simulink model "Glide_slope_controller3"  (R2019b)
settings: Solver=VariableStepAuto  StartTime=0.0  StopTime=400  RelTol=1e-3
values from neighbouring files (symbols this model uses):
  A_gs = A_longitude_lo([1 3 4 2 5], [1 3 4 2 5])    [FindF16Dynamics.m]    (also in FindF16Dynamics_Chapter8.m)
  alpha = 8.49    [FindF16Dynamics.m]    (also in FindF16Dynamics_Chapter8.m = 10.4511; FindF16Dynamics_KIllian.m; trim_F16.m = alpha*pi/180)
  B_gs = A_longitude_lo([1 3 4 2 5], [6, 7])    [FindF16Dynamics.m]    (also in FindF16Dynamics_Chapter8.m)
  C_gs = C_longitude_lo([1 3 4 2 5], [1 3 4 2 5])    [FindF16Dynamics.m]    (also in FindF16Dynamics_Chapter8.m)
  D_gs = D_longitude_lo([1 3 4 2 5], [1])    [FindF16Dynamics.m]    (also in FindF16Dynamics_Chapter8.m = D_longitude_lo([1 3 4 2 5], [1, 2]))
  thrust = 5000    [FindF16Dynamics.m]    (also in FindF16Dynamics_Chapter8.m = 2826.8165; FindF16Dynamics_KIllian.m)
  velocity = 300    [FindF16Dynamics.m]    (also in FindF16Dynamics_Chapter8.m; FindF16Dynamics_KIllian.m = input('Enter the velocity for the simulation (ft/s):  '); FindF16Dynamics_Q6,7.m = 900; FindF16Dynamics_Q6-7.m = 900)
undefined symbols (not defined in the file or in its folder): d_0, Gamma_0, R_0, Slope_Ramp_Gamma, t_flare, tau
libraries: simulink x9
settings Model: Creator=tomas  LastModifiedBy=tomas
settings DebuggingCC: ArithmeticOperatorsInVariantConditions=warning
settings SFSimCC: CustomCodeUndefinedFunction=UseInterfaceOnly

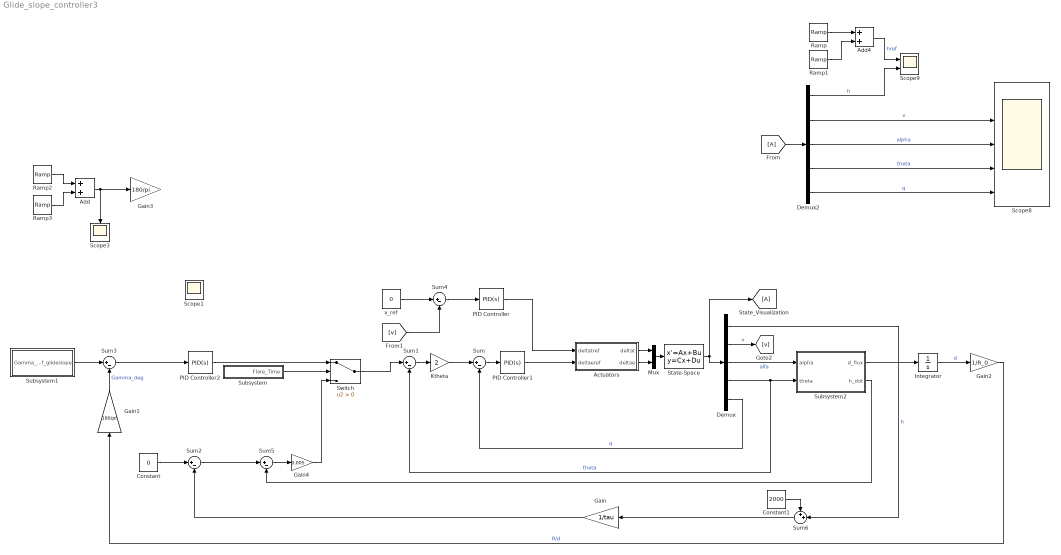
== system Glide_slope_controller3 ==
  Actuators : Subsystem
  Add : Sum
  Add4 : Sum
  Constant : Constant  Value=0
  Constant1 : Constant  Value=2000
  Demux : Demux  Outputs=5
  Demux2 : Demux  Outputs=5
  Gain : Gain  Gain=1/tau
  Gain1 : Gain  Gain=180/pi
  Gain2 : Gain  Gain=1/R_0
  Gain3 : Gain  Gain=180/pi
  Gain4 : Gain  Gain=0.005
  Integrator : Integrator  InitialCondition=d_0
  Ktheta : Gain  Gain=2
  Mux : Mux  Inputs=2
  PID Controller : simulink/Continuous/PID Controller  Controller=PID  Form=Parallel  TimeDomain=Continuous-time  SampleTime=-1  IntegratorMethod=Forward Euler  FilterMethod=Forward Euler  ControllerParametersSource=internal  P=220.313659448083  I=13.48667015583  D=-5.78338115797217  UseFilter=on  N=38.0942658680534  TunerSelectOption=Transfer Function Based (PID Tuner App)  InitialConditionSource=internal  InitialConditionForIntegrator=0  InitialConditionForFilter=0  DifferentiatorICPrevScaledInput=0  ExternalReset=none  TrackingMode=off  Kt=1  LimitOutput=off  UpperSaturationLimit=inf  LowerSaturationLimit=-inf  LinearizeAsGain=on  AntiWindupMode=none  Kb=1  POutMin=[]  POutMax=[]  IOutMin=[]  IOutMax=[]  DOutMin=[]  DOutMax=[]  NOutMin=[]  NOutMax=[]  SumOutMin=[]  SumOutMax=[]  SaturationOutMin=[]  SaturationOutMax=[]  PParamMin=[]  PParamMax=[]  IParamMin=[]  IParamMax=[]  DParamMin=[]  DParamMax=[]  NParamMin=[]  NParamMax=[]  KbParamMin=[]  KbParamMax=[]  KtParamMin=[]  KtParamMax=[]  KbOutMin=[]  KbOutMax=[]  KtOutMin=[]  KtOutMax=[]  IntegratorOutMin=[]  IntegratorOutMax=[]  FilterOutMin=[]  FilterOutMax=[]  SumI1OutMin=[]  SumI1OutMax=[]  SumI2OutMin=[]  SumI2OutMax=[]  SumI3OutMin=[]  SumI3OutMax=[]  SumI4OutMin=[]  SumI4OutMax=[]  SumDOutMin=[]  SumDOutMax=[]  DifferentiatorOutMin=[]  DifferentiatorOutMax=[]  FilterDiffOutCoefMin=[]  FilterDiffOutCoefMax=[]  ReciprocalOutMin=[]  ReciprocalOutMax=[]  SumDenOutMin=[]  SumDenOutMax=[]  SumNumOutMin=[]  SumNumOutMax=[]  DivideOutMin=[]  DivideOutMax=[]  IntegratorContinuousStateAttributes=''  IntegratorStateMustResolveToSignalObject=off  IntegratorRTWStateStorageClass=Auto  FilterContinuousStateAttributes=''  FilterStateMustResolveToSignalObject=off  FilterRTWStateStorageClass=Auto  ParallelPVariant=InternalParameters  IdealPVariant=Disabled  IVariant=InternalParameters  DVariant=InternalParameters  IntegratorVariant=Continuous  SatVariant=Disabled  AWVariant=Passthrough  PCopyVariant=Disabled  TRVariant=Disabled  FdbkBlocksVariant=Forward  IdealPFdbkVariant=Disabled  SatFdbkVariant=Disabled  DerivativeFilterVariant=ContFilter  NVariant=InternalParameters  NCopyVariant=Disabled  FilterICVariant=InternalICsFilter  IntegratorICVariant=InternalICs  ExternalResetVariant=Disabled  TRSumVariant=Passthrough  SumFdbkVariant=Disabled  SumVariant=Sum_PID
  PID Controller1 : simulink/Continuous/PID Controller  Controller=PID  Form=Parallel  TimeDomain=Continuous-time  SampleTime=-1  IntegratorMethod=Forward Euler  FilterMethod=Forward Euler  ControllerParametersSource=internal  P=-5  I=-1  D=-1  UseFilter=on  N=100  TunerSelectOption=Transfer Function Based (PID Tuner App)  InitialConditionSource=internal  InitialConditionForIntegrator=0  InitialConditionForFilter=0  DifferentiatorICPrevScaledInput=0  ExternalReset=none  TrackingMode=off  Kt=1  LimitOutput=off  UpperSaturationLimit=inf  LowerSaturationLimit=-inf  LinearizeAsGain=on  AntiWindupMode=none  Kb=1  POutMin=[]  POutMax=[]  IOutMin=[]  IOutMax=[]  DOutMin=[]  DOutMax=[]  NOutMin=[]  NOutMax=[]  SumOutMin=[]  SumOutMax=[]  SaturationOutMin=[]  SaturationOutMax=[]  PParamMin=[]  PParamMax=[]  IParamMin=[]  IParamMax=[]  DParamMin=[]  DParamMax=[]  NParamMin=[]  NParamMax=[]  KbParamMin=[]  KbParamMax=[]  KtParamMin=[]  KtParamMax=[]  KbOutMin=[]  KbOutMax=[]  KtOutMin=[]  KtOutMax=[]  IntegratorOutMin=[]  IntegratorOutMax=[]  FilterOutMin=[]  FilterOutMax=[]  SumI1OutMin=[]  SumI1OutMax=[]  SumI2OutMin=[]  SumI2OutMax=[]  SumI3OutMin=[]  SumI3OutMax=[]  SumI4OutMin=[]  SumI4OutMax=[]  SumDOutMin=[]  SumDOutMax=[]  DifferentiatorOutMin=[]  DifferentiatorOutMax=[]  FilterDiffOutCoefMin=[]  FilterDiffOutCoefMax=[]  ReciprocalOutMin=[]  ReciprocalOutMax=[]  SumDenOutMin=[]  SumDenOutMax=[]  SumNumOutMin=[]  SumNumOutMax=[]  DivideOutMin=[]  DivideOutMax=[]  IntegratorContinuousStateAttributes=''  IntegratorStateMustResolveToSignalObject=off  IntegratorRTWStateStorageClass=Auto  FilterContinuousStateAttributes=''  FilterStateMustResolveToSignalObject=off  FilterRTWStateStorageClass=Auto  ParallelPVariant=InternalParameters  IdealPVariant=Disabled  IVariant=InternalParameters  DVariant=InternalParameters  IntegratorVariant=Continuous  SatVariant=Disabled  AWVariant=Passthrough  PCopyVariant=Disabled  TRVariant=Disabled  FdbkBlocksVariant=Forward  IdealPFdbkVariant=Disabled  SatFdbkVariant=Disabled  DerivativeFilterVariant=ContFilter  NVariant=InternalParameters  NCopyVariant=Disabled  FilterICVariant=InternalICsFilter  IntegratorICVariant=InternalICs  ExternalResetVariant=Disabled  TRSumVariant=Passthrough  SumFdbkVariant=Disabled  SumVariant=Sum_PID
  PID Controller2 : simulink/Continuous/PID Controller  Controller=PID  Form=Parallel  TimeDomain=Continuous-time  SampleTime=-1  IntegratorMethod=Forward Euler  FilterMethod=Forward Euler  ControllerParametersSource=internal  P=-165.327  I=-1.1958  D=-88.09  UseFilter=on  N=3.0261  TunerSelectOption=Transfer Function Based (PID Tuner App)  InitialConditionSource=internal  InitialConditionForIntegrator=0  InitialConditionForFilter=0  DifferentiatorICPrevScaledInput=0  ExternalReset=none  TrackingMode=off  Kt=1  LimitOutput=off  UpperSaturationLimit=inf  LowerSaturationLimit=-inf  LinearizeAsGain=on  AntiWindupMode=none  Kb=1  POutMin=[]  POutMax=[]  IOutMin=[]  IOutMax=[]  DOutMin=[]  DOutMax=[]  NOutMin=[]  NOutMax=[]  SumOutMin=[]  SumOutMax=[]  SaturationOutMin=[]  SaturationOutMax=[]  PParamMin=[]  PParamMax=[]  IParamMin=[]  IParamMax=[]  DParamMin=[]  DParamMax=[]  NParamMin=[]  NParamMax=[]  KbParamMin=[]  KbParamMax=[]  KtParamMin=[]  KtParamMax=[]  KbOutMin=[]  KbOutMax=[]  KtOutMin=[]  KtOutMax=[]  IntegratorOutMin=[]  IntegratorOutMax=[]  FilterOutMin=[]  FilterOutMax=[]  SumI1OutMin=[]  SumI1OutMax=[]  SumI2OutMin=[]  SumI2OutMax=[]  SumI3OutMin=[]  SumI3OutMax=[]  SumI4OutMin=[]  SumI4OutMax=[]  SumDOutMin=[]  SumDOutMax=[]  DifferentiatorOutMin=[]  DifferentiatorOutMax=[]  FilterDiffOutCoefMin=[]  FilterDiffOutCoefMax=[]  ReciprocalOutMin=[]  ReciprocalOutMax=[]  SumDenOutMin=[]  SumDenOutMax=[]  SumNumOutMin=[]  SumNumOutMax=[]  DivideOutMin=[]  DivideOutMax=[]  IntegratorContinuousStateAttributes=''  IntegratorStateMustResolveToSignalObject=off  IntegratorRTWStateStorageClass=Auto  FilterContinuousStateAttributes=''  FilterStateMustResolveToSignalObject=off  FilterRTWStateStorageClass=Auto  ParallelPVariant=InternalParameters  IdealPVariant=Disabled  IVariant=InternalParameters  DVariant=InternalParameters  IntegratorVariant=Continuous  SatVariant=Disabled  AWVariant=Passthrough  PCopyVariant=Disabled  TRVariant=Disabled  FdbkBlocksVariant=Forward  IdealPFdbkVariant=Disabled  SatFdbkVariant=Disabled  DerivativeFilterVariant=ContFilter  NVariant=InternalParameters  NCopyVariant=Disabled  FilterICVariant=InternalICsFilter  IntegratorICVariant=InternalICs  ExternalResetVariant=Disabled  TRSumVariant=Passthrough  SumFdbkVariant=Disabled  SumVariant=Sum_PID
  Ramp : simulink/Sources/Ramp  slope=-5*pi  start=10  InitialOutput=0
  Ramp1 : simulink/Sources/Ramp  slope=5*pi  start=t_maneuver_1  InitialOutput=0
  Ramp2 : simulink/Sources/Ramp  slope=Slope_Ramp_Gamma  start=0  InitialOutput=Gamma_0
  Ramp3 : simulink/Sources/Ramp  slope=-Slope_Ramp_Gamma  start=t_intercept  InitialOutput=0
  Scope3 : Scope
  Scope8 : Scope  NumInputPorts=5
  Scope9 : Scope  NumInputPorts=2
  State-Space : StateSpace  A=A_gs  B=B_gs  C=C_gs  D=D_gs  InitialCondition=0
  Subsystem : Subsystem
  Subsystem1 : Subsystem
  Subsystem2 : Subsystem
  Sum{,1..5} (6 alike) : Sum  Inputs=|+-
  Sum6 : Sum  Inputs=++|
  Switch : Switch  Criteria=u2 > Threshold
  v_ref : Constant  Value=0
  Scope1 : Scope
  wires:
  State-Space/1 -> Demux/1, [A]
  Demux/5 -> Sum/2  "q"
  Demux2/1 -> Scope9/2  "h"
  Ktheta/1 -> Sum/1
  Sum1/1 -> Ktheta/1
  Integrator/1 -> Gain2/1  "d"
  Mux/1 -> State-Space/1
  Demux/4 -> Subsystem2/2(theta), Sum1/2  "theta"
  Actuators/2(deltae) -> Mux/2
  Actuators/1(deltat) -> Mux/1
  [v] -> Sum4/2
  Gain1/1 -> Sum3/2  "Gamma_deg"
  Ramp/1 -> Add4/1
  Ramp1/1 -> Add4/2
  Add4/1 -> Scope9/1  "href"
  Demux/3 -> Subsystem2/1(alpha)  "alfa"
  Demux/2 -> [v]  "v"
  Gain2/1 -> Gain1/1  "R/d"
  Sum/1 -> PID Controller1/1
  Add/1 -> Scope3/1, Gain3/1
  Ramp2/1 -> Add/1
  Ramp3/1 -> Add/2
  Sum3/1 -> PID Controller2/1
  Sum4/1 -> PID Controller/1
  PID Controller/1 -> Actuators/1(deltatref)
  PID Controller1/1 -> Actuators/2("deltaeref ")
  v_ref/1 -> Sum4/1
  Demux2/2 -> Scope8/2  "v"
  Demux2/3 -> Scope8/3  "alpha"
  Demux2/4 -> Scope8/4  "theta"
  Demux2/5 -> Scope8/5  "q"
  [A] -> Demux2/1
  Subsystem2/1(d_flux) -> Integrator/1
  Gain4/1 -> Switch/3
  Constant/1 -> Sum2/1
  Gain/1 -> Sum2/2
  Subsystem2/2(h_dot) -> Sum5/2
  Sum5/1 -> Gain4/1
  Sum6/1 -> Gain/1
  Subsystem/1(Flare_Time) -> Switch/2
  Sum2/1 -> Sum5/1
  PID Controller2/1 -> Switch/1
  Switch/1 -> Sum1/1
  Constant1/1 -> Sum6/1
  Demux/1 -> Sum6/2  "h"
  Subsystem1/1("Gamma_ref_glideslope ") -> Sum3/1

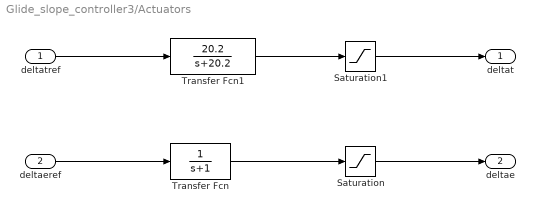
== system Glide_slope_controller3/Actuators ==
  deltatref : Inport
  "deltaeref " : Inport  Port=2
  Saturation : Saturate  UpperLimit=14.5489  LowerLimit=-35.4511
  Saturation1 : Saturate  UpperLimit=19000-thrust  LowerLimit=1000-thrust
  Transfer Fcn : TransferFcn  Denominator=[1 1]
  Transfer Fcn1 : TransferFcn  Numerator=[20.2]  Denominator=[1 20.2]
  deltat : Outport
  deltae : Outport  Port=2
  wires:
  "deltaeref "/1 -> Transfer Fcn/1
  Transfer Fcn/1 -> Saturation/1
  Saturation/1 -> deltae/1
  Saturation1/1 -> deltat/1
  Transfer Fcn1/1 -> Saturation1/1
  deltatref/1 -> Transfer Fcn1/1

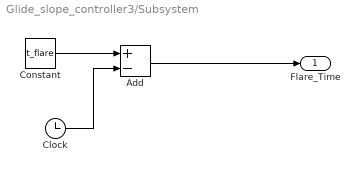
== system Glide_slope_controller3/Subsystem ==
  Add : Sum  Inputs=+-
  Clock : Clock
  Constant : Constant  Value=t_flare
  Flare_Time : Outport
  wires:
  Add/1 -> Flare_Time/1
  Clock/1 -> Add/2
  Constant/1 -> Add/1

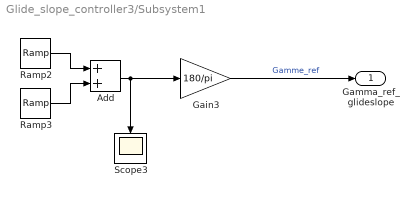
== system Glide_slope_controller3/Subsystem1 ==
  Add : Sum
  Gain3 : Gain  Gain=180/pi
  Ramp2 : simulink/Sources/Ramp  slope=Slope_Ramp_Gamma  start=0  InitialOutput=Gamma_0
  Ramp3 : simulink/Sources/Ramp  slope=-Slope_Ramp_Gamma  start=t_intercept  InitialOutput=0
  Scope3 : Scope
  "Gamma_ref_glideslope " : Outport
  wires:
  Gain3/1 -> "Gamma_ref_glideslope "/1  "Gamme_ref"
  Add/1 -> Scope3/1, Gain3/1
  Ramp2/1 -> Add/1
  Ramp3/1 -> Add/2

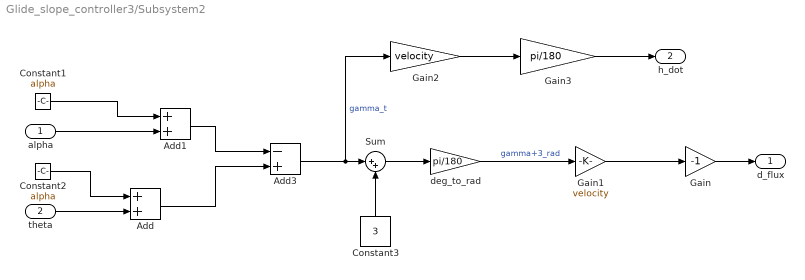
== system Glide_slope_controller3/Subsystem2 ==
  alpha : Inport
  theta : Inport  Port=2
  Add : Sum
  Add1 : Sum
  Add3 : Sum  Inputs=-+
  Constant1 : Constant  Value=alpha
  Constant2 : Constant  Value=alpha
  Constant3 : Constant  Value=3
  Gain : Gain  Gain=-1
  Gain1 : Gain  Gain=velocity
  Gain2 : Gain  Gain=velocity
  Gain3 : Gain  Gain=pi/180
  Sum : Sum  Inputs=|++
  deg_to_rad : Gain  Gain=pi/180
  d_flux : Outport
  h_dot : Outport  Port=2
  wires:
  Constant2/1 -> Add/1
  theta/1 -> Add/2
  Add/1 -> Add3/2
  alpha/1 -> Add1/2
  Constant1/1 -> Add1/1
  Add1/1 -> Add3/1
  Gain/1 -> d_flux/1
  deg_to_rad/1 -> Gain1/1  "gamma+3_rad"
  Gain1/1 -> Gain/1
  Constant3/1 -> Sum/2
  Sum/1 -> deg_to_rad/1
  Add3/1 -> Gain2/1, Sum/1  "gamma_t"
  Gain2/1 -> Gain3/1
  Gain3/1 -> h_dot/1
